simulink model "tanhDistortionSinModel"  (R2019a)
settings: Solver=FixedStepDiscrete  StartTime=0.0  StopTime=inf  RelTol=1e-3
settings Model: Creator=shanewirkes  LastModifiedBy=shanewirkes
settings SolverCC: AutoInsertRateTranBlk=on
settings DataIOCC: LimitDataPoints=on  SaveOutput=off  SignalLogging=off  SaveTime=off
settings OptimizationCC: LifeSpan=inf  SimCompilerOptimization=on
settings DebuggingCC: AlgebraicLoopMsg=error  SingleTaskRateTransMsg=error  AllowSymbolicDim=off  SFUnexpectedBacktrackingDiag=warning  SFNoUnconditionalDefaultTransitionDiag=warning  SFExecutionAtInitializationDiag=none  ArithmeticOperatorsInVariantConditions=warning
settings SFSimCC: SimUseLocalCustomCode=off
settings RTWCC: RTWUseLocalCustomCode=off
settings CodeAppCC: StateflowObjectComments=on
settings GRTTargetCC: TargetLangStandard=C89/C90 (ANSI)  GeneratePreprocessorConditionals=Disable all
settings ConfigComp: CovMetricSettings=dw  CovHtmlReporting=on  CovSaveCumulativeToWorkspaceVar=on  CovSaveSingleToWorkspaceVar=on  CovExternalEMLEnable=off  CovSFcnEnable=off

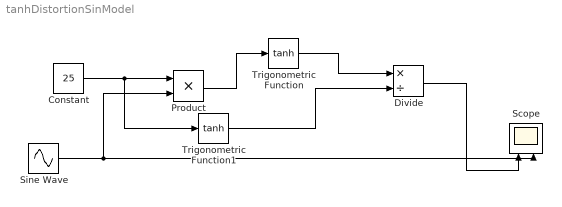
== system tanhDistortionSinModel ==
  Constant : Constant  Value=25
  Divide : Product  Inputs=*/
  Product : Product
  Scope : Scope  NumInputPorts=2
  Sine Wave : Sin  Frequency=4  SampleTime=0
  Trigonometric Function : Trigonometry  Operator=tanh
  Trigonometric Function1 : Trigonometry  Operator=tanh
  wires:
  Sine Wave/1 -> Product/2, Scope/2
  Trigonometric Function/1 -> Divide/1
  Product/1 -> Trigonometric Function/1
  Constant/1 -> Trigonometric Function1/1, Product/1
  Trigonometric Function1/1 -> Divide/2
  Divide/1 -> Scope/1
